simulink library "KSim"  (Simulink 8.3)
settings: Solver=ode45  StartTime=0.0  StopTime=10.0  RelTol=1e-3
undefined symbols (not defined in the file or in its folder): BlueBird_uni_todiff, simiam
settings Model: Creator=jdelacroix  LastModifiedBy=Bird

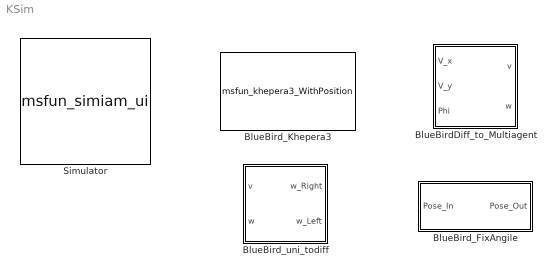
== system KSim ==
  BlueBirdDiff_to_Multiagent : Subsystem  AncestorBlock=simiam/BlueBird_uni_todiff  mask(BlueBird_uni_todiff){l=2}
      mask prompts: l "偏移量（cm）"
      mask help: 这个模块完成自行车模型向机器人模型的转换。
  BlueBird_FixAngile : MATLAB Function  TreatAsAtomicUnit=on
  BlueBird_Khepera3 : M-S-Function  AncestorBlock=simiam/Khepera III  FunctionName=msfun_khepera3_WithPosition  Parameters=x_0,y_0,theta_0,ShowObservation  mask(Khepera3){x_0=0.1, y_0=0.1, theta_0=pi/2, robot_id=1, ShowObservation=on}
      mask prompts: robot_id "ID"; ShowObservation "显示观测"
      mask Display:
      | port_label('output', 1, 'ir_raw')
      | port_label('output', 2, 'wheel_ticks')
      | port_label('output', 3, 'PosFromSim')
      | port_label('output', 4, 'EKF_Out')
      | 
      | port_label('input', 1, 'vel_r')
      | port_label('input', 2, 'vel_l')
  BlueBird_uni_todiff : Subsystem  mask(BlueBird_uni_todiff){r_R=0.0213200003, r_L=0.0213200003, b=0.0896796882}
      mask prompts: r_R "右轮半径（r_R）"; r_L "左轮半径（r_L）"; b "轴距（b）"
      mask help: 这个模块完成自行车模型向机器人模型的转换。
  Simulator : M-S-Function  FunctionName=msfun_simiam_ui  mask(Simulator){}
      mask Display: image(imread('simulink/simiam-round-logo.png'))

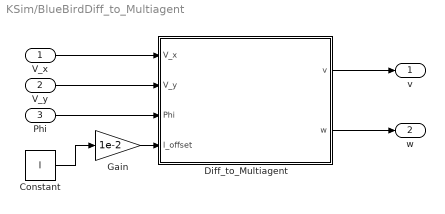
== system KSim/BlueBirdDiff_to_Multiagent ==
  V_x : Inport
  V_y : Inport  Port=2
  Phi : Inport  Port=3
  Constant : Constant  Value=l
  Diff_to_Multiagent : MATLAB Function  TreatAsAtomicUnit=on
  Gain : Gain  Gain=1e-2
  v : Outport
  w : Outport  Port=2
  wires:
  V_x/1 -> Diff_to_Multiagent/1(V_x)
  V_y/1 -> Diff_to_Multiagent/2(V_y)
  Phi/1 -> Diff_to_Multiagent/3(Phi)
  Constant/1 -> Gain/1
  Gain/1 -> Diff_to_Multiagent/4(l_offset)
  Diff_to_Multiagent/1(v) -> v/1
  Diff_to_Multiagent/2(w) -> w/1

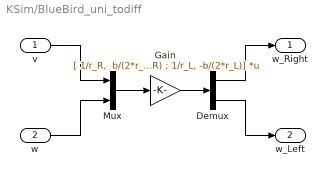
== system KSim/BlueBird_uni_todiff ==
  v : Inport
  w : Inport  Port=2
  Demux : Demux  Outputs=2
  Gain : Gain  Gain="[ 1/r_R,  b/(2*r_R) ; 1/r_L, -b/(2*r_L)]"  Multiplication=Matrix(K*u)
  Mux : Mux  Inputs=2
  w_Right : Outport
  w_Left : Outport  Port=2
  wires:
  w/1 -> Mux/2
  Demux/2 -> w_Left/1
  Gain/1 -> Demux/1
  Demux/1 -> w_Right/1
  v/1 -> Mux/1
  Mux/1 -> Gain/1

== matlab function BlueBirdDiff_to_Multiagent/Diff_to_Multiagent ==
  data: V_x input double; V_y input double; v output double; Phi input double; l_offset input double; w output double
function [v,w] = BlueBird_Diff_to_Multiagent(V_x,V_y,Phi,l_offset)
%#codegen
%l_offset在这个函数里是米
if(l_offset >0)
    Temp = [1 0 ; 0 1/l_offset]*[cos(-Phi) -sin(-Phi); sin(-Phi) cos(-Phi)]*[V_x ; V_y];
    v = Temp(1,1);
    w = Temp(2,1);
else
    v = 0;
    w = 0;
end

== matlab function BlueBird_FixAngile ==
  data: Pose_Out output double; Pose_In input double
function Pose_Out = FixAngile(Pose_In)
%用来修正过大的角度，输入域是：-pi-pi
Rad = Pose_In(3,1);
while (Rad > pi) 
    Rad = Rad - 2 * pi;
end
while (Rad < -pi) 
    Rad = Rad + 2 * pi;
end

Pose_Out = Pose_In;
Pose_Out(3,1) = Rad;
